simulink model "bldc0"  (R2022b)
settings: Solver=ode1  StartTime=0.0  StopTime=0.2  FixedStep=ctrlConst.TsSwitch  MaxStep=1e-6  RelTol=1e-3  EnableMultiTasking=on
values from neighbouring files (symbols this model uses):
  f32_P_AngleCompCur = 5461.0    [bldc.sldd]
  f32_P_AngleCompVol = 1.5    [bldc.sldd]
  f32_P_CurMax_A = 43.0    [bldc.sldd]
  f32_P_DeadPrd = 80.0    [bldc.sldd]
  f32_P_FwcCurMax_A = 54.2    [bldc.sldd]
  f32_P_fwcKi = 0.3    [bldc.sldd]
  f32_P_fwcKp = 11.0    [bldc.sldd]
  f32_P_IdInIF_A = -5.0    [bldc.sldd]
  f32_P_IdKi = 0.00010825    [bldc.sldd]
  f32_P_IdKp = 0.02    [bldc.sldd]
  f32_P_IdqFilter = 1250.0    [bldc.sldd]
  f32_P_IqKi = 0.00010825    [bldc.sldd]
  f32_P_IqKp = 0.02    [bldc.sldd]
  f32_P_MaxTrq_Nm = 1500.0    [bldc.sldd]
  f32_P_MinTrq_Nm = -1500.0    [bldc.sldd]
  f32_P_Modulation = 0.95    [bldc.sldd]
  f32_P_MotorPhi = 0.0026    [bldc.sldd]
  f32_P_PWMFreq = 10000.0    [bldc.sldd]
  f32_P_SpdNegKi = 10.0    [bldc.sldd]
  f32_P_SpdNegKp = 100.0    [bldc.sldd]
  f32_P_SpdNeglimit_rpm = -6000.0    [bldc.sldd]
  f32_P_SpdPosKi = 10.0    [bldc.sldd]
  f32_P_SpdPosKp = 100.0    [bldc.sldd]
  f32_P_SpdPoslimit_rpm = 6000.0    [bldc.sldd]
  f32_P_SpeedKi = 2.5E-6    [bldc.sldd]
  f32_P_SpeedKp = 0.02    [bldc.sldd]
  f32_P_SpeedPiMax = 1.5    [bldc.sldd]
  f32_P_SpeedPiMin = -1.5    [bldc.sldd]
  f32_P_Uqmax = 0.955    [bldc.sldd]
  u16_P_MotorPair = 4.0    [bldc.sldd]
undefined symbols (not defined in the file or in its folder): ECM
libraries: simulink x6, spsabctodq0Lib x1
(part 2 of 2)

== system bldc0/bldc/SVPWM/Switch Case Action Subsystem6 ==
  Action Port : ActionPort  ActionPortLabel=default:
  Constant : Constant  Value=0  OutDataTypeStr=uint32
  Constant1 : Constant  Value=0  OutDataTypeStr=uint32
  Constant2 : Constant  Value=0  OutDataTypeStr=uint32
  Out1 : Outport  VectorParamsAs1DForOutWhenUnconnected=off
  Out2 : Outport  Port=2  VectorParamsAs1DForOutWhenUnconnected=off
  Out3 : Outport  Port=3  VectorParamsAs1DForOutWhenUnconnected=off
  wires:
  Constant2/1 -> Out3/1
  Constant1/1 -> Out2/1
  Constant/1 -> Out1/1

== system bldc0/bldc/Speed Control/Ratelimit ==
  f32_Speedref_rpm : Inport
  f32_SpdLimitPos : Inport  Port=2
  f32_SpdLimitNeg : Inport  Port=3
  Rate Limiter Dynamic : simulink/Discontinuities/Rate Limiter Dynamic
  ref : Outport  VectorParamsAs1DForOutWhenUnconnected=off
  wires:
  f32_Speedref_rpm/1 -> Rate Limiter Dynamic/2
  Rate Limiter Dynamic/1 -> ref/1
  f32_SpdLimitPos/1 -> Rate Limiter Dynamic/1
  f32_SpdLimitNeg/1 -> Rate Limiter Dynamic/3

== system bldc0/bldc/Speed Control/Subsystem ==
  Idfwc : Inport
  Constant : Constant  Value=f32_P_CurMax_A
  Constant1 : Constant  Value=0  OutDataTypeStr=single
  Gain : Gain  Gain=0.5
  Gain1 : Gain  Gain=-1
  Gain2 : Gain  Gain=3*4*f32_P_MotorPhi
  Max : MinMax  Function=max  Inputs=2
  Product : Product
  Product1 : Product
  Sqrt : Sqrt
  Subtract : Sum  Inputs=+-
  max : Outport  VectorParamsAs1DForOutWhenUnconnected=off
  min : Outport  Port=2  VectorParamsAs1DForOutWhenUnconnected=off
  wires:
  Gain1/1 -> min/1
  Sqrt/1 -> Gain2/1
  Max/1 -> Sqrt/1
  Constant1/1 -> Max/1
  Subtract/1 -> Max/2
  Gain/1 -> Subtract/2
  Product1/1 -> Gain/1
  Idfwc/1 -> Product1/2, Product1/1
  Product/1 -> Subtract/1
  Constant/1 -> Product/1, Product/2
  Gain2/1 -> Gain1/1, max/1

== system bldc0/bldc/Speed Control/Subsystem1 ==
  f32_Speedref_rpm : Inport
  f32_SpeedAct_rpm : Inport  Port=2
  Abs : Abs  SaturateOnIntegerOverflow=off
  Constant : Constant  Value=200  OutDataTypeStr=single
  Constant1 : Constant  Value=0.02  OutDataTypeStr=single
  Constant2 : Constant  OutDataTypeStr=single
  Constant4 : Constant  Value=f32_P_SpeedKi
  Gain : Gain  Gain=0.02
  Max : MinMax  Inputs=2
  Product : Product
  Saturation Dynamic : simulink/Discontinuities/Saturation Dynamic  OutMin=[]  OutMax=[]  OutDataTypeStr=Inherit: Same as second input  OutDataType=fixdt(1, 16)  OutScaling=2^-10  DoSatur=off
  Subtract : Sum  Inputs=+-
  Subtract1 : Sum  Inputs=+-
  Ki : Outport
  wires:
  f32_Speedref_rpm/1 -> Subtract/1
  f32_SpeedAct_rpm/1 -> Subtract/2
  Subtract/1 -> Abs/1
  Gain/1 -> Saturation Dynamic/2
  Abs/1 -> Max/2
  Constant/1 -> Subtract1/1, Max/1
  Max/1 -> Subtract1/2
  Subtract1/1 -> Gain/1
  Constant1/1 -> Saturation Dynamic/3
  Constant2/1 -> Saturation Dynamic/1
  Saturation Dynamic/1 -> Product/2
  Constant4/1 -> Product/1
  Product/1 -> Ki/1

== system bldc0/bldc/Torque Control/Ratelimit ==
  f32_TorqueCmd_Nm : Inport
  f32_TrqLimitPos : Inport  Port=2
  f32_TrqLimitNeg : Inport  Port=3
  Rate Limiter Dynamic : simulink/Discontinuities/Rate Limiter Dynamic
  Out1 : Outport  VectorParamsAs1DForOutWhenUnconnected=off
  wires:
  Rate Limiter Dynamic/1 -> Out1/1
  f32_TrqLimitNeg/1 -> Rate Limiter Dynamic/3
  f32_TrqLimitPos/1 -> Rate Limiter Dynamic/1
  f32_TorqueCmd_Nm/1 -> Rate Limiter Dynamic/2

== system bldc0/bldc/Torque Control/SpdNegLimit ==
  f32_SpeedAct_rpm : Inport
  min : Inport  Port=2
  Chart : Stateflow chart  Commented=on  TreatAsAtomicUnit=on
  Constant : Constant  Value=0  OutDataTypeStr=single
  Constant1 : Constant  Value=f32_P_SpdNeglimit_rpm
  Constant2 : Constant  Value=f32_P_SpdNegKp
  Constant3 : Constant  Value=f32_P_SpdNegKi
  MATLAB Function : MATLAB Function  TreatAsAtomicUnit=on
  Unit Delay : UnitDelay  SampleTime=-1  HasFrameUpgradeWarning=on
  out : Outport  VectorParamsAs1DForOutWhenUnconnected=off
  wires:
  MATLAB Function/1(out) -> out/1
  Constant2/1 -> MATLAB Function/3(kp)
  Constant/1 -> MATLAB Function/5(MAX)
  Constant3/1 -> MATLAB Function/4(ki)
  f32_SpeedAct_rpm/1 -> MATLAB Function/2(act)
  min/1 -> MATLAB Function/6(MIN)
  Constant1/1 -> MATLAB Function/1(ref)
  Unit Delay/1 -> MATLAB Function/7("intg ")
  MATLAB Function/2(intg) -> Unit Delay/1

== system bldc0/bldc/Torque Control/SpdPosLimit ==
  f32_SpeedAct_rpm : Inport
  max : Inport  Port=2
  Chart : Stateflow chart  Commented=on  TreatAsAtomicUnit=on
  Constant : Constant  Value=0  OutDataTypeStr=single
  Constant1 : Constant  Value=f32_P_SpdPoslimit_rpm
  Constant4 : Constant  Value=f32_P_SpdPosKp
  Constant5 : Constant  Value=f32_P_SpdPosKi
  MATLAB Function : MATLAB Function  TreatAsAtomicUnit=on
  Unit Delay : UnitDelay  SampleTime=-1  HasFrameUpgradeWarning=on
  out : Outport  VectorParamsAs1DForOutWhenUnconnected=off
  wires:
  max/1 -> MATLAB Function/5(MAX)
  Constant1/1 -> MATLAB Function/1(ref)
  f32_SpeedAct_rpm/1 -> MATLAB Function/2(act)
  Constant4/1 -> MATLAB Function/3(kp)
  Constant5/1 -> MATLAB Function/4(ki)
  MATLAB Function/1(out) -> out/1
  Constant/1 -> MATLAB Function/6(MIN)
  Unit Delay/1 -> MATLAB Function/7("intg ")
  MATLAB Function/2(intg) -> Unit Delay/1

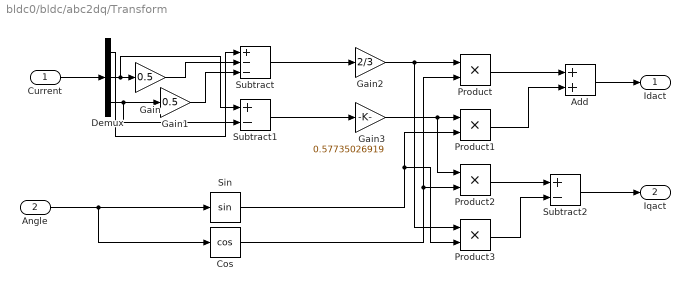
== system bldc0/bldc/abc2dq/Transform ==
  Current : Inport
  Angle : Inport  Port=2
  Add : Sum  OutDataTypeStr=single
  Cos : Trigonometry  Operator=cos  OutputSignalType=real
  Demux : Demux  Outputs=3
  Gain : Gain  Gain=0.5
  Gain1 : Gain  Gain=0.5
  Gain2 : Gain  Gain=2/3
  Gain3 : Gain  Gain=0.57735026919
  Product{,1..3} (4 alike) : Product
  Sin : Trigonometry
  Subtract : Sum  Inputs=+--
  Subtract1 : Sum  Inputs=+-
  Subtract2 : Sum  Inputs=+-  OutDataTypeStr=single
  Idact : Outport
  Iqact : Outport  Port=2
  wires:
  Current/1 -> Demux/1
  Demux/1 -> Subtract/1
  Demux/2 -> Subtract1/1, Gain/1
  Demux/3 -> Subtract1/2, Gain1/1
  Gain/1 -> Subtract/2
  Gain1/1 -> Subtract/3
  Subtract/1 -> Gain2/1
  Subtract1/1 -> Gain3/1
  Gain2/1 -> Product3/1, Product/1
  Cos/1 -> Product2/2, Product/2
  Product/1 -> Add/1
  Gain3/1 -> Product2/1, Product1/1
  Product1/1 -> Add/2
  Add/1 -> Idact/1
  Product2/1 -> Subtract2/1
  Product3/1 -> Subtract2/2
  Subtract2/1 -> Iqact/1
  Angle/1 -> Sin/1, Cos/1
  Sin/1 -> Product3/2, Product1/2

== system bldc0/bldc/abc2dq/filter ==
  Idact : Inport
  Ts : Inport  Port=2
  Constant : Constant  OutDataTypeStr=single
  Constant1 : Constant  Value=f32_P_IdqFilter  OutDataTypeStr=single
  Minus : Sum  Inputs=+-
  Plus : Sum
  Product : Product
  Product1 : Product
  Product2 : Product
  Unit Delay : UnitDelay  SampleTime=-1  HasFrameUpgradeWarning=on
  Outport : Outport
  wires:
  Constant/1 -> Minus/1
  Product2/1 -> Product/1, Minus/2
  Idact/1 -> Product/2
  Product/1 -> Plus/2
  Minus/1 -> Product1/2
  Product1/1 -> Plus/1
  Plus/1 -> Unit Delay/1, Outport/1
  Unit Delay/1 -> Product1/1
  Ts/1 -> Product2/2
  Constant1/1 -> Product2/1

== system bldc0/bldc/abc2dq/filter1 ==
  Iqact : Inport
  Ts : Inport  Port=2
  Constant : Constant  OutDataTypeStr=single
  Constant1 : Constant  Value=f32_P_IdqFilter  OutDataTypeStr=single
  Minus : Sum  Inputs=+-
  Plus : Sum
  Product : Product
  Product1 : Product
  Product2 : Product
  Unit Delay : UnitDelay  SampleTime=-1  HasFrameUpgradeWarning=on
  Outport : Outport
  wires:
  Constant/1 -> Minus/1
  Product2/1 -> Minus/2, Product/1
  Iqact/1 -> Product/2
  Product/1 -> Plus/2
  Minus/1 -> Product1/2
  Product1/1 -> Plus/1
  Plus/1 -> Unit Delay/1, Outport/1
  Unit Delay/1 -> Product1/1
  Constant1/1 -> Product2/1
  Ts/1 -> Product2/2

== matlab function bldc0/bldc/CurrentLoop/MATLAB Function ==
  data: ref input; out output; act input; kp input; ki input; MAX input; MIN input; intg input single; intg output
function [out,intg] = fcn(ref,act,kp,ki,MAX,MIN,intg)
err = ref - act;
temp = err*kp;
out = temp + intg;
if(out>MAX)
    out = MAX;
    if(err<0)
        intg = intg + ki*err;
    end
elseif(out < MIN)
        out = MIN;
        if(err>0)
            intg = intg + ki*err;
        end
else
    intg = intg + ki*err;
end
max(intg,MIN);
min(intg,MAX);

== matlab function bldc0/bldc/CurrentLoop/MATLAB Function1 ==
  data: ref input single; out output single; act input single; kp input single; ki input single; MAX input single; MIN input single; intg input single; intg output
function [out,intg] = fcn(ref,act,kp,ki,MAX,MIN,intg)
err = ref - act;
temp = err*kp;
out = temp + intg;
if(out>MAX)
    out = MAX;
    if(err<0)
        intg = intg + ki*err;
    end
elseif(out < MIN)
        out = MIN;
        if(err>0)
            intg = intg + ki*err;
        end
else
    intg = intg + ki*err;
end
max(intg,MIN);
min(intg,MAX);

== matlab function bldc0/bldc/Torque Control/SpdPosLimit/MATLAB Function ==
  data: ref input; out output; act input; kp input; ki input; MAX input; MIN input; intg input single; intg output
function [out,intg] = fcn(ref,act,kp,ki,MAX,MIN,intg)
err = ref - act;
temp = err*kp;
out = temp + intg;
if(out>MAX)
    out = MAX;
    if(err<0)
        intg = intg + ki*err;
    end
elseif(out < MIN)
        out = MIN;
        if(err>0)
            intg = intg + ki*err;
        end
else
    intg = intg + ki*err;
end
max(intg,MIN);
min(intg,MAX);

== matlab function bldc0/bldc/Torque Control/SpdNegLimit/MATLAB Function ==
  data: ref input; out output; act input; kp input; ki input; MAX input; MIN input; intg input single; intg output
function [out,intg]  = fcn(ref,act,kp,ki,MAX,MIN,intg)
persistent temp;
err = ref - act;
temp = err*kp;
out = temp + intg;
if(out>MAX)
    out = MAX;
    if(err<0)
        intg = intg + ki*err;
    end
elseif(out < MIN)
        out = MIN;
        if(err>0)
            intg = intg + ki*err;
        end
else
    intg = intg + ki*err;
end
max(intg,MIN);
min(intg,MAX);

== stateflow chart bldc0/bldc/CurrentLoop/Ud ==
  state PID
    en:
    err=0;
    integ=0;
    du:
    err=ref-act;
    out=kp*err+integ;
    if out>max
    out=max;
    if(err<0)
    integ=integ+ki*err;
    end
    elseif out<min
    out=min;
    if(err>0)
    integ=integ+ki*err;
    end
    else
    integ=integ+ki*err;
    end
    if integ>max
    integ=max;
    elseif integ <min
    integ=min;
    end
  (default) -> PID
  data: ref input single; act input single; kp input single; ki input single; out output single; integ local single; max input single; min input single; err local single

== matlab function bldc0/bldc/FWC/MATLAB Function1 ==
  data: err input single; out output single; kp input single; ki input single; MAX input single; MIN input single; intg input single; intg output
function [out,intg] = fcn(err,kp,ki,MAX,MIN,intg)
temp = err*kp;
out = temp + intg;
if(out>MAX)
    out = MAX;
    if(err<0)
        intg = intg + ki*err;
    end
elseif(out < MIN)
        out = MIN;
        if(err>0)
            intg = intg + ki*err;
        end
else
    intg = intg + ki*err;
end
max(intg,MIN);
min(intg,MAX);

== stateflow chart bldc0/bldc/CurrentLoop/Uq ==
  state PID
    en:
    err=0;
    integ=0;
    du:
    err=ref-act;
    out=kp*err+integ;
    if out>max
    out=max;
    if(err<0)
    integ=integ+ki*err;
    end
    elseif out<min
    out=min;
    if(err>0)
    integ=integ+ki*err;
    end
    else
    integ=integ+ki*err;
    end
    if integ>max
    integ=max;
    elseif integ <min
    integ=min;
    end
  (default) -> PID
  data: ref input single; act input single; kp input single; ki input single; out output single; integ local single; max input single; min input single; err local single

== stateflow chart bldc0/bldc/Speed Control/Chart ==
  state PID
    en:
    err=0;
    integ=0;
    du:
    err=(ref-act)*0.03192;
    out=kp*err+integ;
    if out>max
    out=max;
    if(err<0)
    integ=integ+ki*err;
    end
    elseif out<min
    out=min;
    if(err>0)
    integ=integ+ki*err;
    end
    else
    integ=integ+ki*err;
    end
    if integ>max
    integ=max;
    elseif integ <min
    integ=min;
    end
  (default) -> PID
  data: ref input single; act input single; kp input single; ki input single; out output single; integ local single; max input single; min input single; err local single

== matlab function bldc0/bldc/Speed Control/MATLAB Function ==
  data: ref input; out output; act input; kp input; ki input; MAX input; MIN input; intgin input single; intgout output
function [out,intgout] = fcn(ref,act,kp,ki,MAX,MIN,intgin)
err = (ref - act)*0.03192;
temp = err*kp;
out = temp + intgin;
if(out>MAX)
    out = MAX;
    if(err<0)
        intgin = intgin + ki*err;
    end
elseif(out < MIN)
        out = MIN;
        if(err>0)
            intgin = intgin + ki*err;
        end
else
    intgin = intgin + ki*err;
end
max(intgin,MIN);
min(intgin,MAX);
intgout = intgin;

== stateflow chart bldc0/bldc/FWC/Chart1 ==
  state PID
    en:
    integ=0;
    du:
    out=kp*err+integ;
    if out>max
    out=max;
    if(err<0)
    integ=integ+ki*err;
    end
    elseif out<min
    out=min;
    if(err>0)
    integ=integ+ki*err;
    end
    else
    integ=integ+ki*err;
    end
    if integ>max
    integ=max;
    elseif integ <min
    integ=min;
    end
  (default) -> PID
  data: err input single; kp input single; ki input single; out output single; integ local single; max input single; min input single; f32_max input single =0.15

== stateflow chart bldc0/bldc/Torque Control/SpdPosLimit/Chart ==
  state PID
    en:
    err=0;
    integ=0;
    du:
    err=ref-act;
    out=kp*err+integ;
    if out>max
    out=max;
    if(err<0)
    integ=integ+ki*err;
    end
    elseif out<min
    out=min;
    if(err>0)
    integ=integ+ki*err;
    end
    else
    integ=integ+ki*err;
    end
    if integ>max
    integ=max;
    elseif integ <min
    integ=min;
    end
  (default) -> PID
  data: ref input single; act input single; kp input single; ki input single; out output single; integ local single; max input single; min input single; err local single

== stateflow chart bldc0/bldc/Torque Control/SpdNegLimit/Chart ==
  state PID
    en:
    err=0;
    integ=0;
    du:
    err=ref-act;
    out=kp*err+integ;
    if out>max
    out=max;
    if(err<0)
    integ=integ+ki*err;
    end
    elseif out<min
    out=min;
    if(err>0)
    integ=integ+ki*err;
    end
    else
    integ=integ+ki*err;
    end
    if integ>max
    integ=max;
    elseif integ <min
    integ=min;
    end
  (default) -> PID
  data: ref input single; act input single; kp input single; ki input single; out output single; integ local single; max input single; min input single; err local single
